simulink model "diagbloque3"  (R2019b)
settings: Solver=VariableStepAuto  StartTime=0.0  StopTime=5  RelTol=1e-3  EnableMultiTasking=on
values from neighbouring files (symbols this model uses):
  ba = 0.001    [TPpelotita.m]
  bp = 1.59    [TPpelotita.m]
  m = 0.0585    [TPpelotita.m]
  r = 0.063/2    (= 0.0315)    [TPpelotita.m]
  v0x = -5    [TPpelotita.m]
  x0 = 15    [TPpelotita.m]
  y0 = 1.5    [TPpelotita.m]
libraries: simulink_extras x2
settings Model: Creator=Paula  LastModifiedBy=Fer
settings DataIOCC: MaxDataPoints=500  ReturnWorkspaceOutputs=off
settings OptimizationCC: LifeSpan=inf
settings DebuggingCC: SFUnexpectedBacktrackingDiag=warning  SFNoUnconditionalDefaultTransitionDiag=warning  ArithmeticOperatorsInVariantConditions=warning
settings SFSimCC: SimUseLocalCustomCode=off  CustomCodeUndefinedFunction=UseInterfaceOnly
settings RTWCC: RTWUseLocalCustomCode=off
settings CodeAppCC: StateflowObjectComments=on
settings GRTTargetCC: TargetLangStandard=C89/C90 (ANSI)  GeneratePreprocessorConditionals=Disable all
settings ConfigComp: CovMetricSettings=dw  CovHtmlReporting=on  CovSaveCumulativeToWorkspaceVar=on  CovSaveSingleToWorkspaceVar=on  CovExternalEMLEnable=off

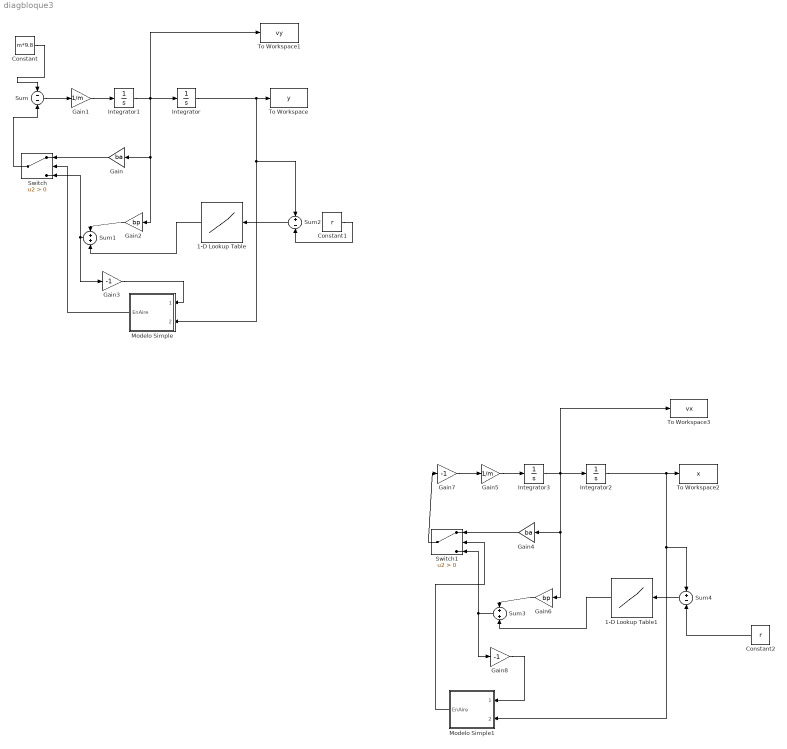
== system diagbloque3 ==
  1-D Lookup Table : Lookup_n-D  NumberOfTableDimensions=1  BreakpointsForDimension1=[0.000152979,0.000299869,0.000439218,0.000573908,0.000701165,0.000827118,0.000954278,0.001083536,0.001209584,0.001340158,0.001478477,0.00161775,0.001752221,0.001887395,0.002024889]  Table=[0.0686,0.4214,1.029,1.8424,3.0282,4.4492,6.0564,7.84,10.241,12.74,14.798,16.905,19.6392,22.344,24.843]  InternalRulePriority=Speed  RndMeth=Simplest  InputSameDT=on
  1-D Lookup Table1 : Lookup_n-D  NumberOfTableDimensions=1  BreakpointsForDimension1=[0.000152979,0.000299869,0.000439218,0.000573908,0.000701165,0.000827118,0.000954278,0.001083536,0.001209584,0.001340158,0.001478477,0.00161775,0.001752221,0.001887395,0.002024889]  Table=[0.0686,0.4214,1.029,1.8424,3.0282,4.4492,6.0564,7.84,10.241,12.74,14.798,16.905,19.6392,22.344,24.843]  InternalRulePriority=Speed  RndMeth=Simplest  InputSameDT=on
  Constant : Constant  Value=m*9.8
  Constant1 : Constant  Value=r
  Constant2 : Constant  Value=r
  Gain : Gain  Gain=ba
  Gain1 : Gain  Gain=1/m
  Gain2 : Gain  Gain=bp
  Gain3 : Gain  Gain=-1
  Gain4 : Gain  Gain=ba
  Gain5 : Gain  Gain=1/m
  Gain6 : Gain  Gain=bp
  Gain7 : Gain  Gain=-1
  Gain8 : Gain  Gain=-1
  Integrator : Integrator  InitialCondition=y0
  Integrator1 : Integrator
  Integrator2 : Integrator  InitialCondition=x0
  Integrator3 : Integrator  InitialCondition=v0x
  Modelo Simple : Subsystem  mask{r=r}
      mask prompts: r "Radio"
      mask help: La salida 'EnAire' es 1 inicialmente. 'EnAire' cambia a 0 cuando la entrada 'Posicion CM' cruza el valor dado por el parametro 'Radio' con tendencia decreciente. Si 'EnAire' es 0, cambiarÃ¡ a 1 cuando 'Fnormal' llegue a 0 con tendencia decreciente.
  Modelo Simple1 : Subsystem  mask{r=r}
      mask prompts: r "Radio"
      mask help: La salida 'EnAire' es 1 inicialmente. 'EnAire' cambia a 0 cuando la entrada 'Posicion CM' cruza el valor dado por el parametro 'Radio' con tendencia decreciente. Si 'EnAire' es 0, cambiarÃ¡ a 1 cuando 'Fnormal' llegue a 0 con tendencia decreciente.
  Sum : Sum  Inputs=--
  Sum1 : Sum
  Sum2 : Sum  Inputs=+-
  Sum3 : Sum
  Sum4 : Sum  Inputs=+-
  Switch : Switch  Criteria=u2 > Threshold
  Switch1 : Switch  Criteria=u2 > Threshold
  To Workspace : ToWorkspace  VariableName=y  SaveFormat=Structure With Time  SampleTime=0.001
  To Workspace1 : ToWorkspace  VariableName=vy  SaveFormat=Structure With Time  SampleTime=0.001
  To Workspace2 : ToWorkspace  VariableName=x  SaveFormat=Structure With Time  SampleTime=0.001
  To Workspace3 : ToWorkspace  VariableName=vx  SaveFormat=Structure With Time  SampleTime=0.001
  wires:
  Switch/1 -> Sum/2
  Gain1/1 -> Integrator1/1
  Integrator1/1 -> To Workspace1/1, Gain2/1, Gain/1, Integrator/1
  Gain/1 -> Switch/1
  Gain2/1 -> Sum1/1
  Sum1/1 -> Switch/3, Gain3/1
  1-D Lookup Table/1 -> Sum1/2
  Constant1/1 -> Sum2/2
  Sum2/1 -> 1-D Lookup Table/1
  Integrator/1 -> Modelo Simple/2(Posicion CM), Sum2/1, To Workspace/1
  Sum/1 -> Gain1/1
  Constant/1 -> Sum/1
  Modelo Simple/1(EnAire) -> Switch/2
  Gain3/1 -> Modelo Simple/1(Fnormal)
  Sum4/1 -> 1-D Lookup Table1/1
  Sum3/1 -> Gain8/1, Switch1/3
  Gain6/1 -> Sum3/1
  Integrator2/1 -> Modelo Simple1/2(Posicion CM), Sum4/1, To Workspace2/1
  1-D Lookup Table1/1 -> Sum3/2
  Integrator3/1 -> To Workspace3/1, Gain6/1, Gain4/1, Integrator2/1
  Gain4/1 -> Switch1/1
  Gain5/1 -> Integrator3/1
  Gain7/1 -> Gain5/1
  Switch1/1 -> Gain7/1
  Constant2/1 -> Sum4/2
  Gain8/1 -> Modelo Simple1/1(Fnormal)
  Modelo Simple1/1(EnAire) -> Switch1/2

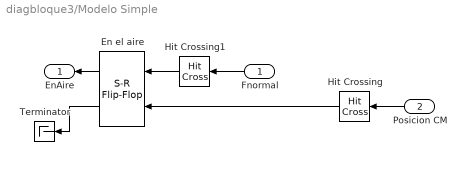
== system diagbloque3/Modelo Simple ==
  Fnormal : Inport
  Posicion CM : Inport  Port=2
  En el aire : simulink_extras/Flip Flops/S-R Flip-Flop  initial_condition=1
  Hit Crossing : HitCross  HitCrossingOffset=r  HitCrossingDirection=falling
  Hit Crossing1 : HitCross  HitCrossingDirection=falling
  Terminator : Terminator
  EnAire : Outport
  wires:
  Hit Crossing1/1 -> En el aire/1
  Hit Crossing/1 -> En el aire/2
  Fnormal/1 -> Hit Crossing1/1
  Posicion CM/1 -> Hit Crossing/1
  En el aire/1 -> EnAire/1
  En el aire/2 -> Terminator/1

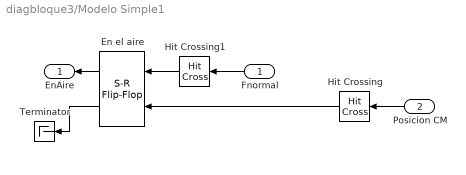
== system diagbloque3/Modelo Simple1 ==
  Fnormal : Inport
  Posicion CM : Inport  Port=2
  En el aire : simulink_extras/Flip Flops/S-R Flip-Flop  initial_condition=1
  Hit Crossing : HitCross  HitCrossingOffset=r  HitCrossingDirection=falling
  Hit Crossing1 : HitCross  HitCrossingDirection=falling
  Terminator : Terminator
  EnAire : Outport
  wires:
  Hit Crossing1/1 -> En el aire/1
  Hit Crossing/1 -> En el aire/2
  Fnormal/1 -> Hit Crossing1/1
  Posicion CM/1 -> Hit Crossing/1
  En el aire/1 -> EnAire/1
  En el aire/2 -> Terminator/1
